simulink model "rigid_body"  (R2023a)
settings: Solver=ode4  StartTime=0.0  StopTime=50  FixedStep=0.01  RelTol=1e-3
values from neighbouring files (symbols this model uses):
  B_vessel = 0    [init_rigid_body.m]
  d_quay = 0    [init_rigid_body.m]
  I = [0.0, 0.0, 0.0]'    [init_rigid_body.m]
  I_added = [0.0, 0.0, 0.0]'    [init_rigid_body.m]
  initial_position = [0,0,0,0,0,0]'    [init_rigid_body.m]
  initial_velocity = [0,0,0,0,0,0]'    [init_rigid_body.m]
  k_quay = 0    [init_rigid_body.m]
  L_vessel = 0    [init_rigid_body.m]
  m = 0.0    (= 0)    [init_rigid_body.m]
  m_added = [0.0, 0.0, 0.0]'    [init_rigid_body.m]
  mu_quay = 0    [init_rigid_body.m]
  quay_1_depth = 0    [init_rigid_body.m]
  quay_1_en = false    [init_rigid_body.m]
  quay_1_p0 = [0, 0]'    [init_rigid_body.m]
  quay_1_p1 = [0, 0]'    [init_rigid_body.m]
  quay_2_depth = 0    [init_rigid_body.m]
  quay_2_en = false    [init_rigid_body.m]
  quay_2_p0 = [0, 0]'    [init_rigid_body.m]
  quay_2_p1 = [0, 0]'    [init_rigid_body.m]
  quay_3_depth = 0    [init_rigid_body.m]
  quay_3_en = false    [init_rigid_body.m]
  quay_3_p0 = [0, 0]'    [init_rigid_body.m]
  quay_3_p1 = [0, 0]'    [init_rigid_body.m]
  quay_4_depth = 0    [init_rigid_body.m]
  quay_4_en = false    [init_rigid_body.m]
  quay_4_p0 = [0, 0]'    [init_rigid_body.m]
  quay_4_p1 = [0, 0]'    [init_rigid_body.m]
libraries: mssSimulink x1
settings Model: Creator=tobiasvt  LastModifiedBy=HalvorPlatou
settings SolverCC: AlgebraicLoopSolver=TrustRegion
settings OptimizationCC: ReuseModelBlockBuffer=off
settings DebuggingCC: UnconnectedInputMsg=warning  UnconnectedOutputMsg=warning  UnconnectedLineMsg=warning
settings ModelReferenceCC: EnableRefExpFcnMdlSchedulingChecks=on
settings SFSimCC: CustomCodeUndefinedFunction=UseInterfaceOnly
settings RTWCC: Description=FMU based on GRT (Functional Mock-up Unit)  SystemTargetFile=grtfmi.tlc  GenerateMakefile=off  TemplateMakefile=none  RetainRTWFile=on  DLArmComputeVersion=19.05
settings STFCustomTargetCC: ConcurrentExecutionCompliant=off  CombineOutputUpdateFcns=on  CodeInterfacePackaging=Reusable function  GRTInterface=off  GenerateAllocFcn=on  UseToolchainInfoCompliant=off  SystemTargetFile=grtfmi.tlc
settings GRTTargetCC: ParMdlRefBuildCompliant=off  CompOptLevelCompliant=off  ConcurrentExecutionCompliant=off  MatFileLogging=off  CodeInterfacePackaging=Reusable function  CPPClassGenCompliant=off  GenerateAllocFcn=on  UseToolchainInfoCompliant=off

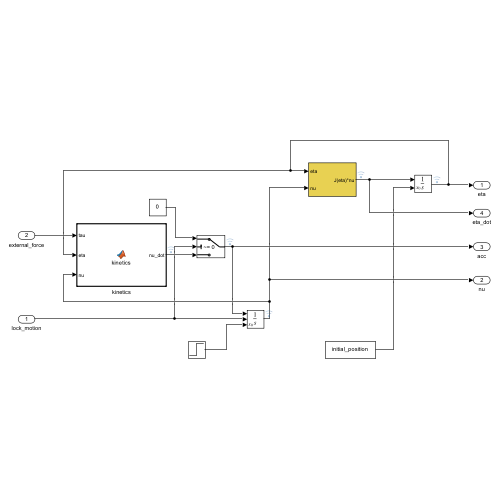
[thumbnail: Simulink's stored preview of the top-level diagram]
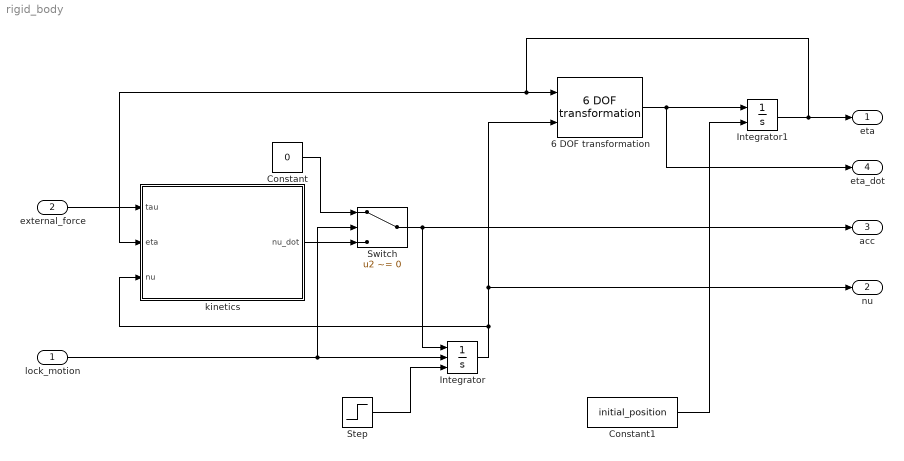
== system rigid_body ==
  lock_motion : Inport  OutDataTypeStr=boolean  PortDimensions=1
  external_force : Inport  Port=2  OutDataTypeStr=double  PortDimensions=6
  6 DOF transformation : mssSimulink/Modelling/Kinematics/6 DOF transformation  SystemSampleTime=-1  VariantActivationTime=update diagram  Latency=0  AutoFrameSizeCalculation=off
  Constant : Constant  Value=0
  Constant1 : Constant  Value=initial_position
  Integrator : Integrator  ExternalReset=level hold  InitialConditionSource=external
  Integrator1 : Integrator  InitialConditionSource=external
  Step : Step  Time=0.1  Before=initial_velocity  After=0  SampleTime=0
  Switch : Switch  Criteria=u2 ~= 0  Threshold=0.5  SaturateOnIntegerOverflow=off  InputSameDT=off
  kinetics : MATLAB Function  TreatAsAtomicUnit=on
  eta : Outport  VectorParamsAs1DForOutWhenUnconnected=off
  nu : Outport  Port=2  VectorParamsAs1DForOutWhenUnconnected=off
  acc : Outport  Port=3  VectorParamsAs1DForOutWhenUnconnected=off
  eta_dot : Outport  Port=4  VectorParamsAs1DForOutWhenUnconnected=off
  wires:
  Integrator1/1 -> 6 DOF transformation/1, kinetics/2(eta), eta/1
  6 DOF transformation/1 -> Integrator1/1, eta_dot/1
  external_force/1 -> kinetics/1(tau)
  Step/1 -> Integrator/3
  Constant1/1 -> Integrator1/2
  lock_motion/1 -> Integrator/2, Switch/2
  Integrator/1 -> kinetics/3(nu), 6 DOF transformation/2, nu/1
  kinetics/1(nu_dot) -> Switch/3
  Switch/1 -> acc/1, Integrator/1
  Constant/1 -> Switch/1

== matlab function rigid_body/kinetics ==
  data: tau input; eta input; nu input; nu_dot output; mu_quay parameter; d_quay parameter; k_quay parameter; B_vessel parameter; L_vessel parameter; quay_1_en parameter boolean; quay_1_depth parameter; quay_1_p1 parameter; quay_1_p0 parameter; quay_2_en parameter boolean; quay_2_depth parameter; quay_2_p1 parameter; quay_2_p0 parameter; quay_3_en parameter boolean; quay_3_depth parameter; quay_3_p1 parameter; quay_3_p0 parameter; quay_4_en parameter boolean; quay_4_depth parameter; quay_4_p1 parameter; quay_4_p0 parameter; m parameter; I parameter; m_added parameter; I_added parameter
function nu_dot  = kinetics(tau, eta, nu, ...
    mu_quay, d_quay, k_quay, B_vessel, L_vessel, ...
    quay_1_en, quay_1_depth, quay_1_p1, quay_1_p0, ...
    quay_2_en, quay_2_depth, quay_2_p1, quay_2_p0, ...
    quay_3_en, quay_3_depth, quay_3_p1, quay_3_p0, ...
    quay_4_en, quay_4_depth, quay_4_p1, quay_4_p0, ...
    m, I, m_added, I_added) ...
%{ 
Simulates a rigid body as a function of external forces, intertia, and a 
collision model between the vessel and the quay(s).

Input variables:
tau     = external forces acting on the vessel (e.g., hydrodynamic forces, control forces, etc.)
eta     = psoe of the vessel (north, east, down, roll, pitch, yaw)
nu      = velocity of the vessel (surge, sway, heave, roll, pitch, yaw)
m       = mass
I       = moment of intertia (roll, pitch, yaw)  All cross-coupling terms neglected
m_added = added mass vector (surge, sway, heave). All cross-coupling terms neglected
I_added = added moment of intertia vector (roll, pitch, yaw). All cross-coupling terms neglected
quay_   = quay model parameters
mu_quay = quay friction coefficient
d_quay  = quay damping coefficient
k_quay  = quay spring coefficient
B_vessel = Vessel width
L_vessel = Vessel lenght

Output:
nu_dot = acceleration
%}

%% Quay collision model
% Setup up the model
num_quays = sum([quay_1_en, quay_2_en, quay_3_en, quay_4_en]);
s         = struct('line', {nan(2, 2)}, 'depth', {nan});
quays     = repmat(s,1,num_quays);

i = 1;

if quay_1_en
    quays(i).line = [reshape(quay_1_p0,2,1), reshape(quay_1_p1,2,1)];
    quays(i).depth = quay_1_depth;
    i = i+1;
end
if quay_2_en
    quays(i).line = [reshape(quay_2_p0,2,1), reshape(quay_2_p1,2,1)];
    quays(i).depth = quay_2_depth;
    i = i+1;
end
if quay_3_en
    quays(i).line = [reshape(quay_3_p0,2,1), reshape(quay_3_p1,2,1)];
    quays(i).depth = quay_3_depth;
    i = i+1;
end
if quay_4_en
    quays(i).line = [reshape(quay_4_p0,2,1), reshape(quay_4_p1,2,1)];
    quays(i).depth = quay_4_depth;
    i = i+1;
end

par.mu = mu_quay;
par.k = k_quay;
par.d = d_quay;
par.v_static = 0.1;
par.stiction_damping = true;
par.vessel_polygon = [
    [ L_vessel/2,  B_vessel/2]
    [ L_vessel/2, -B_vessel/2]
    [-L_vessel/2, -B_vessel/2]
    [-L_vessel/2,  B_vessel/2]
]';

% Calculate forces from quays (ignore vertical forces / moments)
tau_quay = quay_tau(eta, nu, [tau(1), tau(2), 0, 0, 0, tau(6)], quays, par);

%% Construct effective inertia vector

%Inertias
m_effective = zeros(6, 1);
m_effective(1) = m + m_added(1);
m_effective(2) = m + m_added(2);
m_effective(3) = m + m_added(3);
m_effective(4) = I(1) + I_added(1);
m_effective(5) = I(2) + I_added(2);
m_effective(6) = I(3) + I_added(3);

%% Construct Coriolis force vector
C = zeros(6, 6);

C(1, 6) = -m_effective(2) * nu(2);
C(2, 6) =  m_effective(1) * nu(1);

tau_coriolis = -C * nu;

%% Calculate acceleration integration

tau_total = tau + tau_quay + tau_coriolis;

nu_dot = zeros(6, 1);

for i =1:6
    if (m_effective(i) ~= 0.0) % Avoid calculating accelerations if any inertia component is zero
        nu_dot(i) = tau_total(i) / m_effective(i);
    end
end
end
